simulink model "parent_model"  (Simulink 8.3)
settings: Solver=ode3  StartTime=0.0  StopTime=10.0  RelTol=1e-3
libraries: test_library x5, sub_library x2
settings Model: Creator=ladmin  LastModifiedBy=ladmin
settings OptimizationCC: InlineParams=on
settings DebuggingCC: MultiTaskDSMMsg=warning  MultiTaskCondExecSysMsg=none  StateNameClashWarn=none  StrictBusMsg=None
settings RTWCC: IncludeERTFirstTime=on
settings GRTTargetCC: CombineOutputUpdateFcns=on  GRTInterface=off

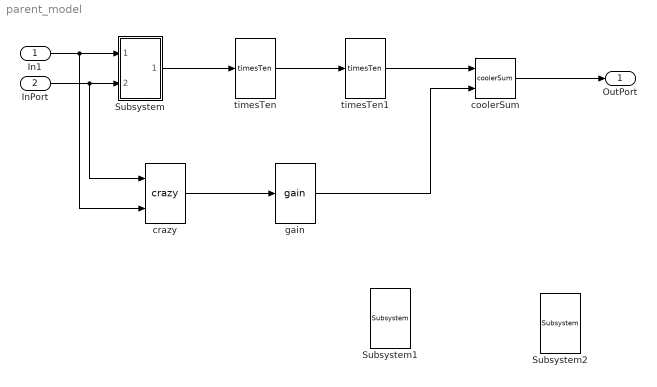
== system parent_model ==
  In1 : Inport
  InPort : Inport  Port=2  mask(TL_Inport){data={'date',735866.65645377315}}
      settings: CopyFcn=if exist('tl_reset_reviewflag') == 2, tl_reset_reviewflag(gcbh); end  DeleteFcn=if exist('delete_tlblock','file')==2,delete_tlblock(gcbh);end  NameChangeFcn=if exist('rename_tlblock','file')==2,rename_tlblock(gcbh);end  OpenFcn=if exist('tl_open_blockdlg','file')==2,tl_open_blockdlg(gcbh);else,open_system(gcbh,'parameter');end
      mask Help: eval(['if exist(''tl_online_help'',''file'') == 2, tl_online_help(''Topic'',''TL_Inport''),else, web([''jar:file:///'',matlabroot,''/help/toolbox/simulink/help.jar!/slref/' lower(get_param(gcbh,'Blocktype')) '.html''], ''-helpbrowser''),end'])
      mask Display: plot([0.2 0.35 NaN 0.65 0.8],[0 1 NaN 0 1]);
  Subsystem : Subsystem
  Subsystem1 : sub_library/Subsystem
  Subsystem2 : sub_library/Subsystem
  coolerSum : test_library/coolerSum  data={'date',735866.66384885414}
  crazy : test_library/crazy
  gain : test_library/crazy/gain
  timesTen : test_library/timesTen
  timesTen1 : test_library/timesTen
  OutPort : Outport  mask(TL_Outport){data={'date',735866.65739972226}}
      settings: CopyFcn=if exist('tl_reset_reviewflag') == 2, tl_reset_reviewflag(gcbh); end  DeleteFcn=if exist('delete_tlblock','file')==2,delete_tlblock(gcbh);end  NameChangeFcn=if exist('rename_tlblock','file')==2,rename_tlblock(gcbh);end  OpenFcn=if exist('tl_open_blockdlg','file')==2,tl_open_blockdlg(gcbh);else,open_system(gcbh,'parameter');end
      mask Help: eval(['if exist(''tl_online_help'',''file'') == 2, tl_online_help(''Topic'',''TL_Outport''),else, web([''jar:file:///'',matlabroot,''/help/toolbox/simulink/help.jar!/slref/' lower(get_param(gcbh,'Blocktype')) '.html''], ''-helpbrowser''),end'])
      mask Display: plot([0.2 0.35 NaN 0.65 0.8],[0 1 NaN 0 1]);
  wires:
  In1/1 -> crazy/2, Subsystem/1(In1)
  Subsystem/1(Out1) -> timesTen/1
  timesTen/1 -> timesTen1/1
  timesTen1/1 -> coolerSum/1
  crazy/1 -> gain/1
  InPort/1 -> crazy/1, Subsystem/2(In2)
  coolerSum/1 -> OutPort/1
  gain/1 -> coolerSum/2

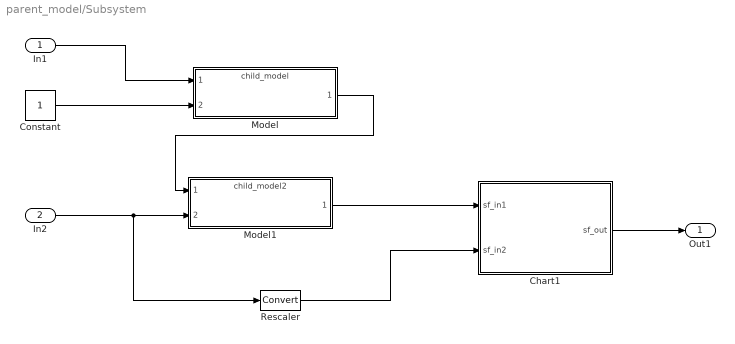
== system parent_model/Subsystem ==
  In1 : Inport
  In2 : Inport  Port=2
  Chart1 : Stateflow chart  TreatAsAtomicUnit=on
  Constant : Constant
  Model : ModelReference  ModelNameDialog=child_model.slx  SimulationMode=Normal  ModelReferenceVersion=1.2  CopyOfModelName=child_model.slx  DefaultDataLogging=on
  Model1 : ModelReference  ModelNameDialog=child_model2.slx  SimulationMode=Normal  ModelReferenceVersion=1.8  CopyOfModelName=child_model2.slx  DefaultDataLogging=on
  Rescaler : DataTypeConversion  mask(TL_Rescaler){data={'date',735866.64311961806}}
      settings: DeleteFcn=if exist('delete_tlblock','file')==2,delete_tlblock(gcbh);end  NameChangeFcn=if exist('rename_tlblock','file')==2,rename_tlblock(gcbh);end  OpenFcn=if exist('tl_open_blockdlg','file')==2,tl_open_blockdlg(gcbh);else,open_system(gcbh,'parameter');end
      mask Help: eval(['if exist(''tl_online_help'',''file'') == 2, tl_online_help(''Topic'',''TL_Rescaler''),else, web([''jar:file:///'',matlabroot,''/help/toolbox/simulink/help.jar!/slref/' lower(get_param(gcbh,'Blocktype')) '.html''], ''-helpbrowser''),end'])
      mask Display: plot([-0.05, 1.05, NaN, -0.05, 1.05],[.01, .01, NaN, .99, .99])
  Out1 : Outport
  wires:
  In1/1 -> Model/1
  Model/1 -> Model1/1
  Constant/1 -> Model/2
  Model1/1 -> Chart1/1(sf_in1)
  In2/1 -> Rescaler/1, Model1/2
  Chart1/1(sf_out) -> Out1/1
  Rescaler/1 -> Chart1/2(sf_in2)

== stateflow chart Subsystem/Chart1 ==
  state entry:
    sf_out = 10
  data: sf_in1 input double; sf_in2 input double; sf_out output double
